simulink model "PWM_module"  (R2015b)
settings: Solver=VariableStepAuto  StartTime=0.0  StopTime=10.0  RelTol=1e-3
libraries: powerlib x12
settings Model: Creator=shangwei  LastModifiedBy=root

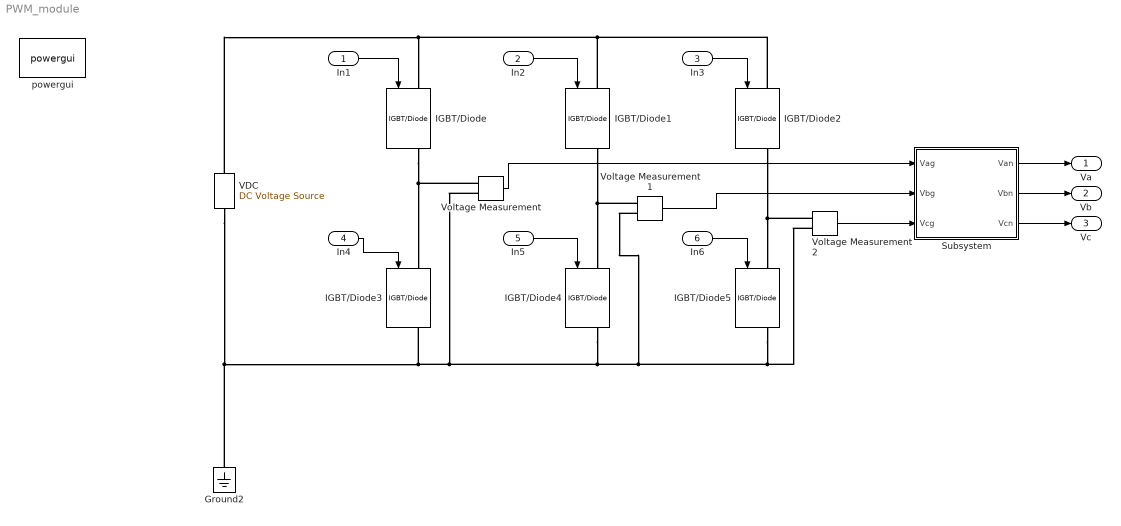
== system PWM_module ==
  In1 : Inport
  In2 : Inport  Port=2
  In3 : Inport  Port=3
  In4 : Inport  Port=4
  In5 : Inport  Port=5
  In6 : Inport  Port=6
  Ground2 : powerlib/Elements/Ground  LConnTagsString=a
  IGBT/Diode{,1..5} (6 alike) : powerlib/Power Electronics/IGBT//Diode  Ron=1e-3  Rs=1e5  Cs=inf  Measurements=on
  Subsystem : Subsystem
  VDC : powerlib/Electrical Sources/DC Voltage Source  Amplitude=24  Measurements=Voltage
  Voltage Measurement : powerlib/Measurements/Voltage Measurement  PhasorSimulation=off  OutputType=Complex  PSBequivalent=0
  Voltage Measurement1 : powerlib/Measurements/Voltage Measurement  PhasorSimulation=off  OutputType=Complex  PSBequivalent=0
  Voltage Measurement2 : powerlib/Measurements/Voltage Measurement  PhasorSimulation=off  OutputType=Complex  PSBequivalent=0
  powergui : powerlib/powergui  Priority=1  SimulationMode=Continuous  SolverType=Tustin/Backward Euler (TBE)  SampleTime=50e-6  frequency=60  SPID=off  DisableSnubberDevices=off  DisableRonSwitches=off  DisableVfSwitches=off  SwTol=0  DisplayEquations=off  Interpol=off  ExternalGateDelay=off  methode=off  Ts=10  FunctionMessages=off  echomessages=off  HookPort=off  EnableUseOfTLC=off  x0status=blocks  frequencyindice=0  Pbase=100e6  ErrMax=1e-4  Iterations=50  UnitsV=kV  UnitsW=MW  buscounter=0  RestoreLinks=warning  ResistiveCurrentMeasurement=off  Frange=[0:2:500]  Ylog=off  Xlog=on  ShowGrid=off  save=off  variable=ZData  structure=0  ZoomFFT=off  StartTime=0.0  cycles=1  DisplayStyle=1  fundamental=60  FreqAxis=off  MaxFrequency=1000  frequencyindicesteady=1  RmsSteady=1  display=off
  Va : Outport
  Vb : Outport  Port=2
  Vc : Outport  Port=3
  wires:
  In1/1 -> IGBT/Diode/1
  In2/1 -> IGBT/Diode1/1
  In3/1 -> IGBT/Diode2/1
  In4/1 -> IGBT/Diode3/1
  In5/1 -> IGBT/Diode4/1
  In6/1 -> IGBT/Diode5/1
  Voltage Measurement/1 -> Subsystem/1(Vag)
  Voltage Measurement1/1 -> Subsystem/2(Vbg)
  Voltage Measurement2/1 -> Subsystem/3(Vcg)
  Subsystem/1(Van) -> Va/1
  Subsystem/2(Vbn) -> Vb/1
  Subsystem/3(Vcn) -> Vc/1
  connections:
  IGBT/Diode/RConn1 -- Voltage Measurement/LConn1 -- IGBT/Diode3/LConn1
  IGBT/Diode1/RConn1 -- Voltage Measurement1/LConn1 -- IGBT/Diode4/LConn1
  IGBT/Diode2/RConn1 -- Voltage Measurement2/LConn1 -- IGBT/Diode5/LConn1
  VDC/RConn1 -- IGBT/Diode2/LConn1 -- IGBT/Diode1/LConn1 -- IGBT/Diode/LConn1
  VDC/LConn1 -- Ground2/LConn1 -- IGBT/Diode3/RConn1 -- Voltage Measurement/LConn2 -- IGBT/Diode4/RConn1 -- Voltage Measurement2/LConn2 -- IGBT/Diode5/RConn1 -- Voltage Measurement1/LConn2

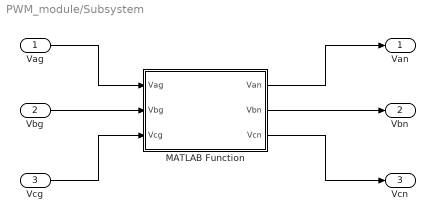
== system PWM_module/Subsystem ==
  Vag : Inport
  Vbg : Inport  Port=2
  Vcg : Inport  Port=3
  MATLAB Function : MATLAB Function  TreatAsAtomicUnit=on
  Van : Outport
  Vbn : Outport  Port=2
  Vcn : Outport  Port=3
  wires:
  Vag/1 -> MATLAB Function/1(Vag)
  Vbg/1 -> MATLAB Function/2(Vbg)
  Vcg/1 -> MATLAB Function/3(Vcg)
  MATLAB Function/1(Van) -> Van/1
  MATLAB Function/2(Vbn) -> Vbn/1
  MATLAB Function/3(Vcn) -> Vcn/1

== matlab function PWM_module/Subsystem/MATLAB Function ==
  data: Vag input; Van output; Vbg input; Vcg input; Vbn output; Vcn output
function [Van, Vbn, Vcn] = poletophase(Vag, Vbg, Vcg)
%#codegen
Trans = [ 2/3 -1/3 -1/3 ; -1/3 2/3 -1/3 ; -1/3 -1/3 2/3];

u = [Vag; Vbg; Vcg];
y = Trans * u ;
Van = y(1);
Vbn = y(2);
Vcn = y(3);
